simulink model "Hand_Dryer_Controller_Model"  (R2025b)
settings: Solver=FixedStepDiscrete  StartTime=0.0  StopTime=inf  FixedStep=0.001  MaxStep=1  RelTol=1e-3
settings Model: Creator=rkash  LastModifiedBy=rkash

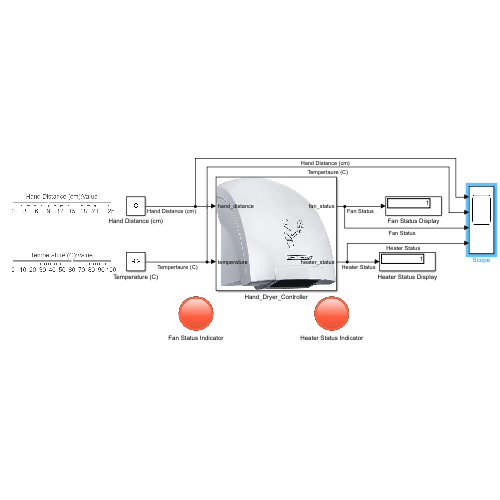
[thumbnail: Simulink's stored preview of the top-level diagram]
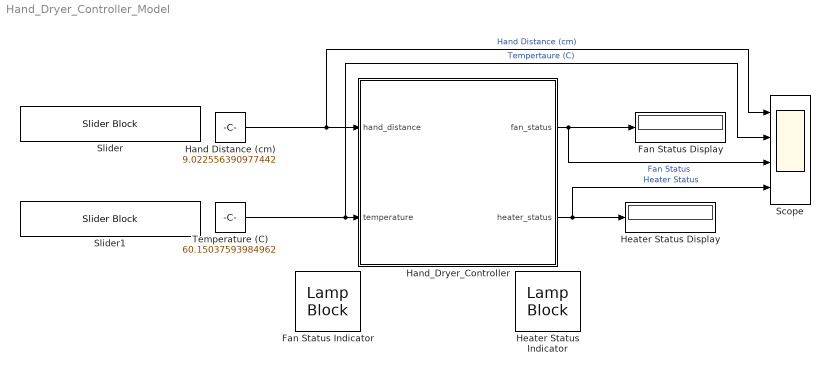
== system Hand_Dryer_Controller_Model ==
  Fan Status Display : Display
  Fan Status Indicator : LampBlock  LabelPosition=Hide  DefaultColor=[19.0, 159.0, 255.0]
  Hand Distance (cm) : Constant  Value=9.022556390977442
  Hand_Dryer_Controller : Stateflow chart  TreatAsAtomicUnit=on
  Heater Status Display : Display
  Heater Status Indicator : LampBlock  LabelPosition=Hide  DefaultColor=[19.0, 159.0, 255.0]
  Scope : Scope  NumInputPorts=4
      settings: ActiveDisplayYMinimum=8.25358851674641  ActiveDisplayYMaximum=15.94326725905673
  Slider : SliderBlock  ScaleMax=25
  Slider1 : SliderBlock
  Temperature (C) : Constant  Value=60.15037593984962
  wires:
  Hand Distance (cm)/1 -> Scope/1, Hand_Dryer_Controller/1(hand_distance)  "Hand Distance (cm)"
  Temperature (C)/1 -> Scope/2, Hand_Dryer_Controller/2(temperature)  "Tempertaure (C)"
  Hand_Dryer_Controller/1(fan_status) -> Fan Status Display/1, Scope/3  "Fan Status"
  Hand_Dryer_Controller/2(heater_status) -> Scope/4, Heater Status Display/1  "Heater Status"

== stateflow chart Hand_Dryer_Controller_Model/Hand_Dryer_Controller ==
  state Fan_State_Logic [parallel]
    en: fan_status = boolean(0);
    settings: executionOrder=1
    state Fan_Status_OFF
      en: fan_status = boolean(0);
    state Hand_Removal_Check
    state Hand_Presence_Check
    state Fan_Status_ON
      en: fan_status = boolean(1);
    (default) -> Fan_Status_OFF
    Fan_Status_ON -> Fan_Status_OFF [order 1] : [after(max_run_time, sec)]
    Hand_Presence_Check -> Fan_Status_OFF [order 2] : [hand_distance >= hand_near_threshold]
    Hand_Removal_Check -> Fan_Status_OFF [order 1] : [after(hand_removal_time ,sec) && hand_distance > hand_far_threshold ]
    Fan_Status_OFF -> Hand_Presence_Check : [hand_distance < hand_near_threshold ]
    Hand_Removal_Check -> Fan_Status_ON [order 2] : [hand_distance <= hand_far_threshold]
    Fan_Status_ON -> Hand_Removal_Check [order 2] : [hand_distance > hand_far_threshold]
    Hand_Presence_Check -> Fan_Status_ON [order 1] : [after(hand_presence_time, sec) && hand_distance < hand_near_threshold]
  state Heater_State_Logic [parallel]
    en: heater_status = boolean(0);
    settings: executionOrder=2
    state Heater_Status_OFF
      en: heater_status = boolean(0);
    state Heater_Status_ON
      en: heater_status = boolean(1);
    (default) -> Heater_Status_OFF
    Heater_Status_ON -> Heater_Status_OFF : [fan_status == 0 || temperature >= heater_off_temp]
    Heater_Status_OFF -> Heater_Status_ON : [fan_status == 1 && temperature < heater_on_temp]
  data: hand_distance input; temperature input; fan_status output; heater_status output; hand_presence_time local =1; hand_removal_time local =3; hand_near_threshold local =10; hand_far_threshold local =15; max_run_time local =60; heater_off_temp local =70; heater_on_temp local =65
